simulink model "problem_5_6_1_simulink"  (R2017b)
settings: Solver=VariableStepAuto  StartTime=0.0  StopTime=3  RelTol=1e-3
undefined symbols (not defined in the file or in its folder): DiscIntNeverNeededParam
settings Model: Creator=ghost  LastModifiedBy=ghost

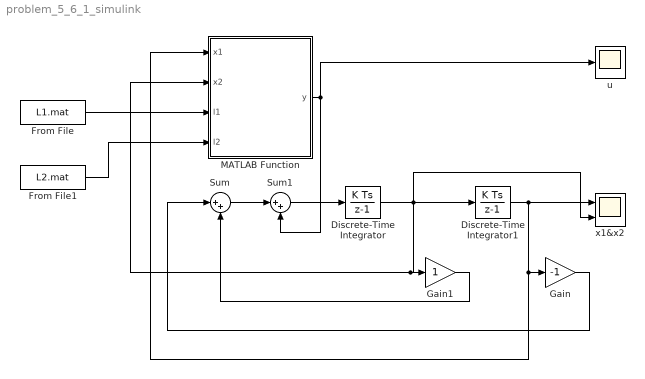
== system problem_5_6_1_simulink ==
  Discrete-Time Integrator : DiscreteIntegrator  InitialCondition=2  InitialConditionSetting=State (most efficient)  ICPrevOutput=DiscIntNeverNeededParam  ICPrevScaledInput=DiscIntNeverNeededParam
  Discrete-Time Integrator1 : DiscreteIntegrator  InitialCondition=1  InitialConditionSetting=State (most efficient)  ICPrevOutput=DiscIntNeverNeededParam  ICPrevScaledInput=DiscIntNeverNeededParam
  From File : FromFile  FileName=L1.mat  SampleTime=0
  From File1 : FromFile  FileName=L2.mat  SampleTime=0
  Gain : Gain  Gain=-1
  Gain1 : Gain
  MATLAB Function : MATLAB Function  TreatAsAtomicUnit=on
  Sum : Sum  Inputs=|++
  Sum1 : Sum  Inputs=|++
  u : Scope
  x1&x2 : Scope  NumInputPorts=2
  wires:
  Discrete-Time Integrator/1 -> x1&x2/2, MATLAB Function/2(x2), Gain1/1, Discrete-Time Integrator1/1
  Discrete-Time Integrator1/1 -> x1&x2/1, MATLAB Function/1(x1), Gain/1
  Gain1/1 -> Sum/2
  Gain/1 -> Sum/1
  From File/1 -> MATLAB Function/3(l1)
  From File1/1 -> MATLAB Function/4(l2)
  Sum/1 -> Sum1/1
  Sum1/1 -> Discrete-Time Integrator/1
  MATLAB Function/1(y) -> u/1, Sum1/2

== matlab function problem_5_6_1_simulink/MATLAB Function ==
  data: x1 input; y output; x2 input; l1 input; l2 input
function y = get_u(x1, x2, l1, l2)

X = [ x1, x2 ]
L = [ l1, l2 ]
y = -L * transpose(X);
